simulink model "Assignment2_3K04"  (R2022b)
settings: Solver=VariableStepAuto  StartTime=0.0  StopTime=10.0  RelTol=1e-3
libraries: frdmk64flib x5, etargetslib x2
settings Model: Creator=Venka  LastModifiedBy=Venka

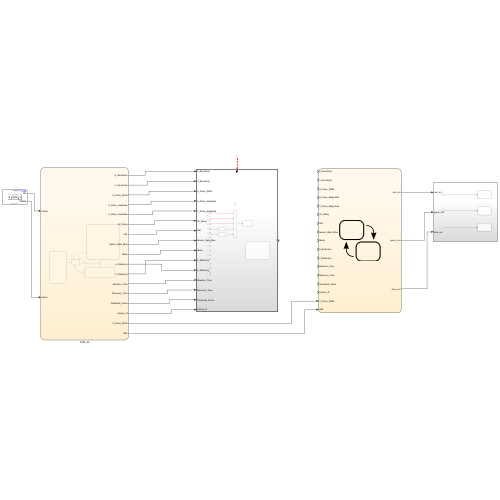
[thumbnail: Simulink's stored preview of the top-level diagram]
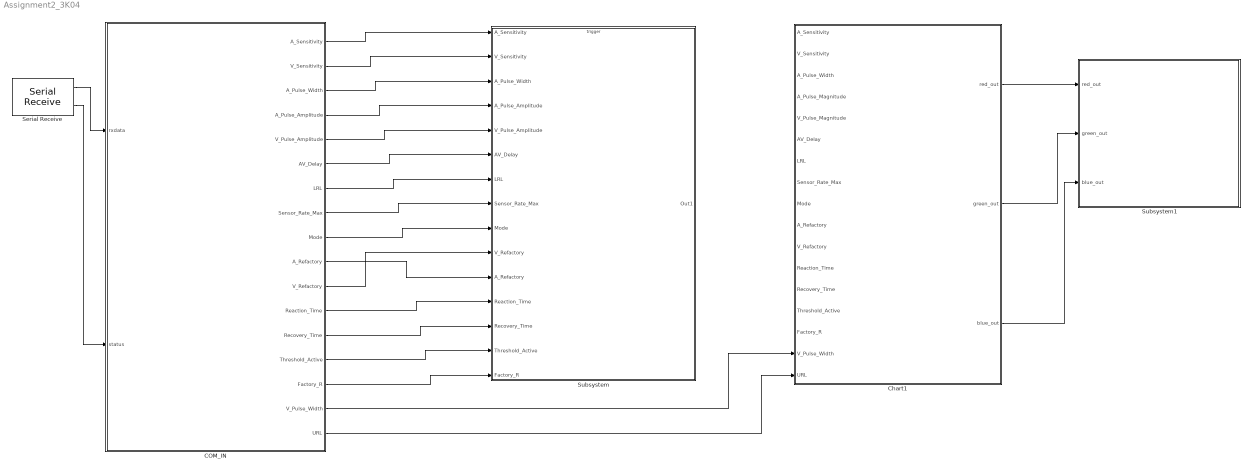
== system Assignment2_3K04 ==
  COM_IN : Stateflow chart  TreatAsAtomicUnit=on
      settings: PortSchema="{\"entries\":[{\"content\":{\"sides\":[{\"content\":{\"connectorIds\":[\"In1\",\"In2\"]},\"type\":\"ConnectorPlacement.EquallySpacedRectSide\",\"uuid\":\"1ea119dc-cb00-4fad-82d7-196495d224c1\"},{\"content\":{\"connectorIds\":[\"Out1\",\"Out2\",\"Out3\",\"Out5\",\"Out6\",\"Out7\",\"Out8\",\"Out10\",\"Out11\",\"Out16\",\"Out17\",\"Out12\",\"Out13\",\"Out14\",\"Out15\",\"Out4\",\"Out9\"],\"side\":\"RIGHT\"},\"type\":\"ConnectorPlacement.EquallySpacedRectSide\",\"uuid\":\"f449a325-17e5-4499-9ff5-f8bdb5edca51\"},{\"content\":{\"connectorIds\":[],\"side\":\"TOP\"},\"type\":\"ConnectorPlacement.EquallySpacedRectSide\",\"uuid\":\"a745425d-949a-4fc0-8c63-370e8ec96d73\"}]},\"type\":\"ConnectorPlacement.EquallySpacedConnector\",\"uuid\":\"62797f9e-adfc-4e87-9d12-3d7822b0a8ae\"}],\"packageUris\":[\"http://schema.mathworks.com/mf0/Connector/R2020b\"],\"version\":\"1.0\"}"
  Chart1 : Stateflow chart  TreatAsAtomicUnit=on
      settings: PortSchema="{\"entries\":[{\"content\":{\"sides\":[{\"content\":{\"connectorIds\":[\"In1\",\"In2\",\"In3\",\"In5\",\"In6\",\"In7\",\"In8\",\"In11\",\"In10\",\"In16\",\"In17\",\"In12\",\"In13\",\"In14\",\"In15\",\"In4\",\"In9\"]},\"type\":\"ConnectorPlacement.EquallySpacedRectSide\",\"uuid\":\"9009545e-9c08-48b8-88cc-47c57c0df39c\"},{\"content\":{\"connectorIds\":[\"Out1\",\"Out2\",\"Out3\"],\"side\":\"RIGHT\"},\"type\":\"ConnectorPlacement.EquallySpacedRectSide\",\"uuid\":\"307c9463-9cd3-4b6f-8cbf-f0c48cd358a8\"},{\"content\":{\"connectorIds\":[],\"side\":\"TOP\"},\"type\":\"ConnectorPlacement.EquallySpacedRectSide\",\"uuid\":\"acac19c5-529d-4f6b-ba79-95b7a159a1df\"}]},\"type\":\"ConnectorPlacement.EquallySpacedConnector\",\"uuid\":\"54b50964-4a86-4b0a-ab76-f2e426866175\"}],\"packageUris\":[\"http://schema.mathworks.com/mf0/Connector/R2020b\"],\"version\":\"1.0\"}"
  Serial Receive : frdmk64flib/Serial Receive  SCIModule=0  Baudrate=uint32(9600)  Parity=None  StopBits=1  HardwareFlowControl=None  ByteOrder=LittleEndian  DataType=uint8  DataLength=10  BlockingMode=off  OutputStatus=on  SampleTime=0.1
  Subsystem : Subsystem
  Subsystem1 : Subsystem
  wires:
  Serial Receive/1 -> COM_IN/1(rxdata)
  Serial Receive/2 -> COM_IN/2(status)
  COM_IN/1(A_Sensitivity) -> Subsystem/1(A_Sensitivity)
  COM_IN/9(URL) -> Chart1/9(URL)
  COM_IN/6(V_Pulse_Amplitude) -> Subsystem/5(V_Pulse_Amplitude)
  COM_IN/5(A_Pulse_Amplitude) -> Subsystem/4(A_Pulse_Amplitude)
  COM_IN/4(V_Pulse_Width) -> Chart1/4(V_Pulse_Width)
  Chart1/1(red_out) -> Subsystem1/1(red_out)
  Chart1/3(blue_out) -> Subsystem1/3(blue_out)
  Chart1/2(green_out) -> Subsystem1/2(green_out)
  ? -> Subsystem/Trigger
  COM_IN/3(A_Pulse_Width) -> Subsystem/3(A_Pulse_Width)
  COM_IN/8(LRL) -> Subsystem/7(LRL)
  COM_IN/7(AV_Delay) -> Subsystem/6(AV_Delay)
  COM_IN/2(V_Sensitivity) -> Subsystem/2(V_Sensitivity)
  COM_IN/10(Sensor_Rate_Max) -> Subsystem/8(Sensor_Rate_Max)
  COM_IN/16(A_Refactory) -> Subsystem/11(A_Refactory)
  COM_IN/11(Mode) -> Subsystem/9(Mode)
  COM_IN/12(Reaction_Time) -> Subsystem/12(Reaction_Time)
  COM_IN/13(Recovery_Time) -> Subsystem/13(Recovery_Time)
  COM_IN/14(Threshold_Active) -> Subsystem/14(Threshold_Active)
  COM_IN/15(Factory_R) -> Subsystem/15(Factory_R)
  COM_IN/17(V_Refactory) -> Subsystem/10(V_Refactory)

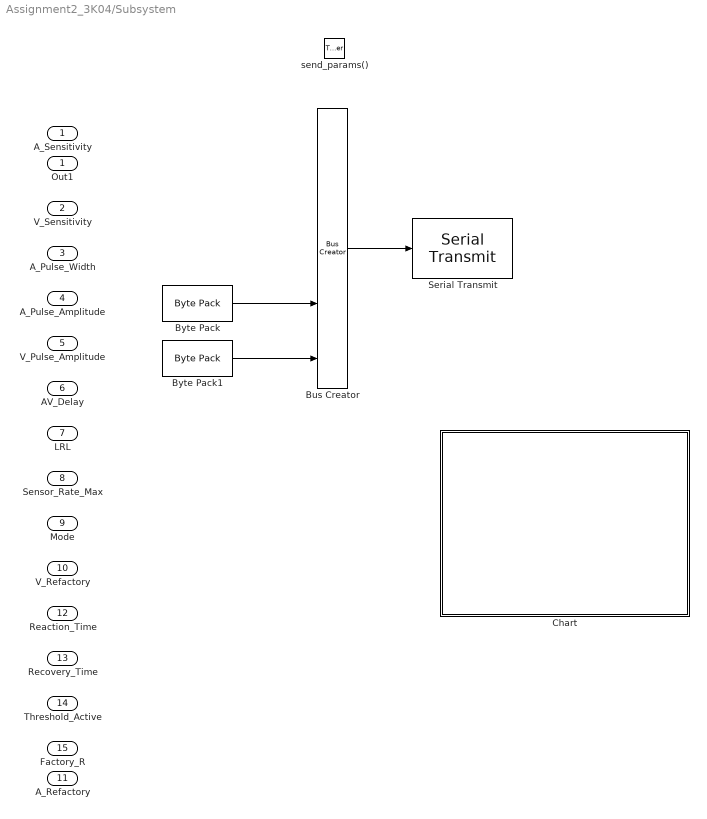
== system Assignment2_3K04/Subsystem ==
  A_Sensitivity : Inport
  V_Sensitivity : Inport  Port=2
  A_Pulse_Width : Inport  Port=3
  A_Pulse_Amplitude : Inport  Port=4
  V_Pulse_Amplitude : Inport  Port=5
  AV_Delay : Inport  Port=6
  LRL : Inport  Port=7
  Sensor_Rate_Max : Inport  Port=8
  Mode : Inport  Port=9
  V_Refactory : Inport  Port=10
  A_Refactory : Inport  Port=11
  Reaction_Time : Inport  Port=12
  Recovery_Time : Inport  Port=13
  Threshold_Active : Inport  Port=14
  Factory_R : Inport  Port=15
  send_params() : TriggerPort  IsSimulinkFunction=on  FunctionName=send_params  FunctionVisibility=port  VariantControl=(inherit)  PortDimensions=1
  Bus Creator : BusCreator  Inputs=5
  Byte Pack : etargetslib/Byte Pack  datatypes={'double'}  byteAlign=1
  Byte Pack1 : etargetslib/Byte Pack  datatypes={'double'}  byteAlign=1
  Chart : Stateflow chart  TreatAsAtomicUnit=on
  Serial Transmit : frdmk64flib/Serial Transmit  SCIModule=0  Baudrate=uint32(9600)  Parity=None  StopBits=1  HardwareFlowControl=None  ByteOrder=LittleEndian  BlockingMode=on  OutputStatus=off
  Out1 : Outport
  wires:
  ? -> Bus Creator/1
  ? -> Bus Creator/2
  ? -> Bus Creator/3
  ? -> Byte Pack/1
  ? -> Byte Pack1/1
  Byte Pack/1 -> Bus Creator/4
  Byte Pack1/1 -> Bus Creator/5
  Bus Creator/1 -> Serial Transmit/1

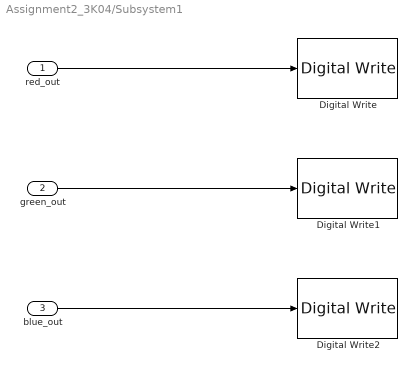
== system Assignment2_3K04/Subsystem1 ==
  red_out : Inport
  green_out : Inport  Port=2
  blue_out : Inport  Port=3
  Digital Write : frdmk64flib/Digital Write  Whichpin=RED_LED
  Digital Write1 : frdmk64flib/Digital Write  Whichpin=GREEN_LED
  Digital Write2 : frdmk64flib/Digital Write  Whichpin=BLUE_LED
  wires:
  red_out/1 -> Digital Write/1
  green_out/1 -> Digital Write1/1
  blue_out/1 -> Digital Write2/1

== stateflow chart Assignment2_3K04/COM_IN ==
  settings: executeAtInitialization=1
  state SET_PARAM
    entry:
    MODE=cast(rxdata(1),'uint16');
    LRL=cast(rxdata(2),'uint16');
    URL=cast(rxdata(3),'uint16');
    MAX_SENSOR_Rate=cast(rxdata(4),'uint16');
    AV_Delay=cast(rxdata(5),'uint16');
    Volt_A_Pulse_Amplitude=typecast(rxdata(6:13),'double');
    Volt_V_Pulse_Amplitude=typecast(rxdata(14:21),'double');
    A_Pulse_Width=cast(rxdata(22),'uint16');
    V_Pulse_Width=cast(rxdata(23),'uint16');
    Volt_A_Sensitivity=typecast(rxdata(24:31),'double');
    Volt_V_Sensitivity=typecast(rxdata(32:39),'double');
    V_Refractory_Period=typecast(rxdata(40:41),'uint16');
    A_Refractory_Period=typecast(rxdata(42:43),'uint16');
    PVARP=cast(rxdata(44),'uint16');
    Rate_Smoothing=cast(rxdata(45),'uint16');
    Activity_Threshold=typecast(rxdata(46:53),'double');
    Reaction_Time=cast(rxdata(54),'uint16');
    Response_Factor=cast(rxdata(55),'double');
    Recovery_Time=cast(rxdata(56),'uint16');
    LRL_Period = 60000/cast(LRL,'uint16')
    LEDR=1;
    LEDB=0;
  state INITIAL
    entry:
    LRL=60;
    URL=50;
    MAX_SENSOR_Rate=0;
    AV_Delay=20;
    Volt_A_Pulse_Amplitude=4;
    Volt_V_Pulse_Amplitude=4;
    A_Pulse_Width=10;
    V_Pulse_Width=10;
    Volt_A_Sensitivity=4;
    Volt_V_Sensitivity=4;
    V_Refractory_Period=300;
    A_Refractory_Period=300;
    PVARP=0;
    Rate_Smoothing=0;
    Activity_Threshold=0.1;
    Reaction_Time=10;
    Response_Factor=10;
    Recovery_Time=10;
    LRL_Period=10;
    MODE=1;
  state STANDBY
  state ECHO_PARAM
    entry:
    send_params();
    LEDB=1;
    LEDR=0;
  (default) -> INITIAL
  SET_PARAM -> STANDBY
  (junction 7) -> STANDBY [order 2]
  (junction 8) -> SET_PARAM [order 1] : [rxdata(57) == hex2dec('00')]
  INITIAL -> STANDBY
  (junction 7) -> (junction 8) [order 1]
  STANDBY -> (junction 7) : [status == 0]
  (junction 8) -> ECHO_PARAM [order 2] : [rxdata(57) == hex2dec('01')]
  ECHO_PARAM -> STANDBY
  data: rxdata input; status input; A_Sensitivity output; V_Sensitivity output; A_Pulse_Width output; V_Pulse_Width output; A_Pulse_Amplitude output; V_Pulse_Amplitude output; AV_Delay output; LRL output; URL output; Sensor_Rate_Max output; Mode output; Reaction_Time output; Recovery_Time output; Threshold_Active output; Factory_R output; A_Refactory output; V_Refactory output

== stateflow chart Assignment2_3K04/Chart1 ==
  data: A_Sensitivity input; V_Sensitivity input; A_Pulse_Width input; V_Pulse_Width input; A_Pulse_Magnitude input; V_Pulse_Magnitude input; AV_Delay input; LRL input; URL input; Mode input; red_out output; green_out output; blue_out output; Sensor_Rate_Max input; Reaction_Time input; Recovery_Time input; Threshold_Active input; Factory_R input; A_Refactory input; V_Refactory input

== stateflow chart Assignment2_3K04/Subsystem/Chart ==
  state OFF
    entry:
    red_out = 0;
    green_out = 0;
    blue_out = 0;
  state RED_ON
    entry:
    red_out = 1;
    green_out = 0;
    blue_out = 0;
  state BLUE_ON
    entry:
    red_out = 0;
    green_out = 0;
    blue_out = 1;
  state GREEN_ON
    entry:
    red_out = 0;
    green_out = 1;
    blue_out = 0;
  state Activity_Rate
  state Up
    entry:
    Time = 0;
    during:
    Adapted_Rate = Response_Factor*(Time/Reaction_Time)/(1+(Time/Reaction_Time)*(Response_Factor-1))*Activity_Rate + LRL;
    Time = Time + 1/1000;
    exit:
    Time = 0;
  state Max
    entry:
    Adapted_Rate = Max_Sensor_Rate;
  state Down
    entry:
    Time = 0;
    Rate_Diff = Adapted_Rate - LRL;
    during:
    Adapted_Rate = Adapted_Rate - (Rate_Diff/Recovery_Time)*Time;
    Time = Time + 1/1000;
    exit:
    Time = 0;
  state Start
    entry:
    Adapted_Rate = LRL;
  state Min
  (default) -> OFF [order 1]
  OFF -> (junction 11) : after(off_time, sec)
  (junction 11) -> RED_ON [order 1] : [red_enable==1]
  (junction 11) -> (junction 9) [order 2]
  (junction 7) -> OFF
  RED_ON -> (junction 9) : after(switch_time, msec)
  (junction 9) -> GREEN_ON [order 1] : [green_enable == 1]
  (junction 3) -> (junction 7) [order 1]
  BLUE_ON -> (junction 7) : after(switch_time, msec)
  (junction 9) -> (junction 3) [order 2]
  GREEN_ON -> (junction 3) : after(switch_time, msec)
  (junction 3) -> BLUE_ON [order 2] : [blue_enable== 1]
  Up -> Activity_Rate [order 2] : [Adapted_Rate>=Activity_Rate+LRL]
  Up -> Up [order 3] : [Time >= Reaction_Time]{Time = 0}
  Activity_Rate -> Down [order 2] : [Activity < Activity_Threshold]
  Activity_Rate -> Up [order 1] : [Activity >= Activity_Threshold]
  Up -> Max [order 1] : [Adapted_Rate >= Max_Sensor_Rate]
  Min -> Up : [Activity >= Activity_Threshold]
  Max -> Down : [Activity < Activity_Threshold]
  Up -> Down [order 4] : [Activity < Activity_Threshold]
  Down -> Up [order 1] : [Activity >= Activity_Threshold]
  (default) -> Start [order 2]
  Start -> Down
  Down -> Min [order 2] : [Adapted_Rate == LRL]
  Down -> Down [order 3] : [Time >= Recovery_Time]{Time = 0}
